simulink model "sm_dump_trailer"  (R2021b)
settings: Solver=VariableStepAuto  StartTime=0.0  StopTime=10  FixedStep=0.0001  RelTol=1e-3  AbsTol=1e-3  EnableMultiTasking=on
model workspace: external: MATLAB File sm_dump_trailer_params.m (data not in the file)
undefined symbols (not defined in the file or in its folder): base, bed, cylinder, lowerarm, sigbuilder_block, upperarm, X, Y, Z
libraries: sm_lib x65, sm_dump_trailer_lib x20, fl_lib x7, nesl_utility x4, simulink x4, sm_interface_elements_lib x1
(part 2 of 3)

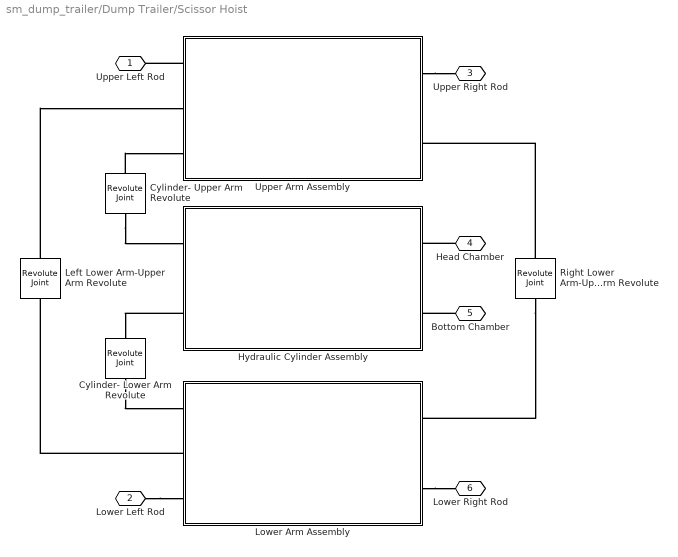
== system sm_dump_trailer/Dump Trailer/Scissor Hoist ==
  Cylinder- Lower Arm Revolute : sm_lib/Joints/Revolute Joint  JointMode=Normal  SenseConstraintForce=off  SenseConstraintForceX=off  SenseConstraintForceY=off  SenseConstraintForceZ=off  SenseConstraintTorque=off  SenseConstraintTorqueX=off  SenseConstraintTorqueY=off  SenseConstraintTorqueZ=off  SenseTotalForce=off  SenseTotalForceX=off  SenseTotalForceY=off  SenseTotalForceZ=off  SenseTotalTorque=off  SenseTotalTorqueX=off  SenseTotalTorqueY=off  SenseTotalTorqueZ=off  CompositeWrenchDir=FollowerOnBase  CompositeWrenchFrame=BaseFrame  EquilibriumPosition=0  EquilibriumPositionUnits=deg  SpringStiffness=0  SpringStiffnessUnits=N*m/deg  DampingCoefficient=0  DampingCoefficientUnits=N*m/(deg/s)  TorqueActuationMode=NoTorque  MotionActuationMode=ComputedMotion  SensePosition=off  SenseVelocity=off  SenseAcceleration=off  SenseTorqueForce=off  SenseLowerLimitTorqueForce=off  SenseUpperLimitTorqueForce=off  LowerLimitSpecify=off  LowerLimitBound=-90  LowerLimitBoundUnits=deg  LowerLimitStiffness=1e4  LowerLimitStiffnessUnits=N*m/deg  LowerLimitDamping=10  LowerLimitDampingUnits=N*m/(deg/s)  LowerLimitTransitionRegionWidth=0.1  LowerLimitTransitionRegionWidthUnits=deg  UpperLimitSpecify=off  UpperLimitBound=90  UpperLimitBoundUnits=deg  UpperLimitStiffness=1e4  UpperLimitStiffnessUnits=N*m/deg  UpperLimitDamping=10  UpperLimitDampingUnits=N*m/(deg/s)  UpperLimitTransitionRegionWidth=0.1  UpperLimitTransitionRegionWidthUnits=deg  PositionTargetSpecify=off  PositionTargetPriority=High  PositionTargetValue=0  PositionTargetValueUnits=deg  VelocityTargetSpecify=off  VelocityTargetPriority=High  VelocityTargetValue=0  VelocityTargetValueUnits=deg/s
  Cylinder- Upper Arm Revolute : sm_lib/Joints/Revolute Joint  JointMode=Normal  SenseConstraintForce=off  SenseConstraintForceX=off  SenseConstraintForceY=off  SenseConstraintForceZ=off  SenseConstraintTorque=off  SenseConstraintTorqueX=off  SenseConstraintTorqueY=off  SenseConstraintTorqueZ=off  SenseTotalForce=off  SenseTotalForceX=off  SenseTotalForceY=off  SenseTotalForceZ=off  SenseTotalTorque=off  SenseTotalTorqueX=off  SenseTotalTorqueY=off  SenseTotalTorqueZ=off  CompositeWrenchDir=FollowerOnBase  CompositeWrenchFrame=BaseFrame  EquilibriumPosition=0  EquilibriumPositionUnits=deg  SpringStiffness=0  SpringStiffnessUnits=N*m/deg  DampingCoefficient=0  DampingCoefficientUnits=N*m/(deg/s)  TorqueActuationMode=NoTorque  MotionActuationMode=ComputedMotion  SensePosition=off  SenseVelocity=off  SenseAcceleration=off  SenseTorqueForce=off  SenseLowerLimitTorqueForce=off  SenseUpperLimitTorqueForce=off  LowerLimitSpecify=off  LowerLimitBound=-90  LowerLimitBoundUnits=deg  LowerLimitStiffness=1e4  LowerLimitStiffnessUnits=N*m/deg  LowerLimitDamping=10  LowerLimitDampingUnits=N*m/(deg/s)  LowerLimitTransitionRegionWidth=0.1  LowerLimitTransitionRegionWidthUnits=deg  UpperLimitSpecify=off  UpperLimitBound=90  UpperLimitBoundUnits=deg  UpperLimitStiffness=1e4  UpperLimitStiffnessUnits=N*m/deg  UpperLimitDamping=10  UpperLimitDampingUnits=N*m/(deg/s)  UpperLimitTransitionRegionWidth=0.1  UpperLimitTransitionRegionWidthUnits=deg  PositionTargetSpecify=off  PositionTargetPriority=High  PositionTargetValue=0  PositionTargetValueUnits=deg  VelocityTargetSpecify=off  VelocityTargetPriority=High  VelocityTargetValue=0  VelocityTargetValueUnits=deg/s
  Hydraulic Cylinder Assembly : Subsystem
      mask Display: image(fullfile(matlabroot,'toolbox','physmod','sm','smdemos','dump_trailer','images','sm_dump_trailer_hydraulic_cylinder_assembly.png'));
  Left Lower Arm-Upper Arm Revolute : sm_lib/Joints/Revolute Joint  JointMode=Normal  SenseConstraintForce=off  SenseConstraintForceX=off  SenseConstraintForceY=off  SenseConstraintForceZ=off  SenseConstraintTorque=off  SenseConstraintTorqueX=off  SenseConstraintTorqueY=off  SenseConstraintTorqueZ=off  SenseTotalForce=off  SenseTotalForceX=off  SenseTotalForceY=off  SenseTotalForceZ=off  SenseTotalTorque=off  SenseTotalTorqueX=off  SenseTotalTorqueY=off  SenseTotalTorqueZ=off  CompositeWrenchDir=FollowerOnBase  CompositeWrenchFrame=BaseFrame  EquilibriumPosition=0  EquilibriumPositionUnits=deg  SpringStiffness=0  SpringStiffnessUnits=N*m/deg  DampingCoefficient=0  DampingCoefficientUnits=N*m/(deg/s)  TorqueActuationMode=NoTorque  MotionActuationMode=ComputedMotion  SensePosition=off  SenseVelocity=off  SenseAcceleration=off  SenseTorqueForce=off  SenseLowerLimitTorqueForce=off  SenseUpperLimitTorqueForce=off  LowerLimitSpecify=off  LowerLimitBound=-90  LowerLimitBoundUnits=deg  LowerLimitStiffness=1e4  LowerLimitStiffnessUnits=N*m/deg  LowerLimitDamping=10  LowerLimitDampingUnits=N*m/(deg/s)  LowerLimitTransitionRegionWidth=0.1  LowerLimitTransitionRegionWidthUnits=deg  UpperLimitSpecify=off  UpperLimitBound=90  UpperLimitBoundUnits=deg  UpperLimitStiffness=1e4  UpperLimitStiffnessUnits=N*m/deg  UpperLimitDamping=10  UpperLimitDampingUnits=N*m/(deg/s)  UpperLimitTransitionRegionWidth=0.1  UpperLimitTransitionRegionWidthUnits=deg  PositionTargetSpecify=off  PositionTargetPriority=High  PositionTargetValue=0  PositionTargetValueUnits=deg  VelocityTargetSpecify=off  VelocityTargetPriority=High  VelocityTargetValue=0  VelocityTargetValueUnits=deg/s
  Lower Arm Assembly : Subsystem
      mask Display: image(fullfile(matlabroot,'toolbox','physmod','sm','smdemos','dump_trailer','images','sm_dump_trailer_lower_arm_assembly.png'));
  Right Lower Arm-Upper Arm Revolute : sm_lib/Joints/Revolute Joint  JointMode=Normal  SenseConstraintForce=off  SenseConstraintForceX=off  SenseConstraintForceY=off  SenseConstraintForceZ=off  SenseConstraintTorque=off  SenseConstraintTorqueX=off  SenseConstraintTorqueY=off  SenseConstraintTorqueZ=off  SenseTotalForce=off  SenseTotalForceX=off  SenseTotalForceY=off  SenseTotalForceZ=off  SenseTotalTorque=off  SenseTotalTorqueX=off  SenseTotalTorqueY=off  SenseTotalTorqueZ=off  CompositeWrenchDir=FollowerOnBase  CompositeWrenchFrame=BaseFrame  EquilibriumPosition=0  EquilibriumPositionUnits=deg  SpringStiffness=0  SpringStiffnessUnits=N*m/deg  DampingCoefficient=0  DampingCoefficientUnits=N*m/(deg/s)  TorqueActuationMode=NoTorque  MotionActuationMode=ComputedMotion  SensePosition=off  SenseVelocity=off  SenseAcceleration=off  SenseTorqueForce=off  SenseLowerLimitTorqueForce=off  SenseUpperLimitTorqueForce=off  LowerLimitSpecify=off  LowerLimitBound=-90  LowerLimitBoundUnits=deg  LowerLimitStiffness=1e4  LowerLimitStiffnessUnits=N*m/deg  LowerLimitDamping=10  LowerLimitDampingUnits=N*m/(deg/s)  LowerLimitTransitionRegionWidth=0.1  LowerLimitTransitionRegionWidthUnits=deg  UpperLimitSpecify=off  UpperLimitBound=90  UpperLimitBoundUnits=deg  UpperLimitStiffness=1e4  UpperLimitStiffnessUnits=N*m/deg  UpperLimitDamping=10  UpperLimitDampingUnits=N*m/(deg/s)  UpperLimitTransitionRegionWidth=0.1  UpperLimitTransitionRegionWidthUnits=deg  PositionTargetSpecify=off  PositionTargetPriority=High  PositionTargetValue=0  PositionTargetValueUnits=deg  VelocityTargetSpecify=off  VelocityTargetPriority=High  VelocityTargetValue=0  VelocityTargetValueUnits=deg/s
  Upper Arm Assembly : Subsystem
      mask Display: image(fullfile(matlabroot,'toolbox','physmod','sm','smdemos','dump_trailer','images','sm_dump_trailer_upper_arm_assembly.png'));
  Upper Left Rod : PMIOPort  Side=Left
  Lower Left Rod : PMIOPort  Port=2  Side=Left
  Upper Right Rod : PMIOPort  Port=3  Side=Right
  Head Chamber : PMIOPort  Port=4  Side=Right
  Bottom Chamber : PMIOPort  Port=5  Side=Right
  Lower Right Rod : PMIOPort  Port=6  Side=Right
  connections:
  Right Lower Arm-Upper Arm Revolute/LConn1 -- Lower Arm Assembly/RConn1
  Lower Arm Assembly/LConn2 -- Left Lower Arm-Upper Arm Revolute/LConn1
  Upper Arm Assembly/LConn1 -- Upper Left Rod/RConn1
  Upper Arm Assembly/RConn1 -- Upper Right Rod/RConn1
  Lower Arm Assembly/RConn2 -- Lower Right Rod/RConn1
  Left Lower Arm-Upper Arm Revolute/RConn1 -- Upper Arm Assembly/LConn2
  Right Lower Arm-Upper Arm Revolute/RConn1 -- Upper Arm Assembly/RConn2
  Lower Left Rod/RConn1 -- Lower Arm Assembly/LConn3
  Head Chamber/RConn1 -- Hydraulic Cylinder Assembly/RConn1
  Bottom Chamber/RConn1 -- Hydraulic Cylinder Assembly/RConn2
  Cylinder- Lower Arm Revolute/LConn1 -- Lower Arm Assembly/LConn1
  Hydraulic Cylinder Assembly/LConn2 -- Cylinder- Lower Arm Revolute/RConn1
  Cylinder- Upper Arm Revolute/LConn1 -- Hydraulic Cylinder Assembly/LConn1
  Cylinder- Upper Arm Revolute/RConn1 -- Upper Arm Assembly/LConn3

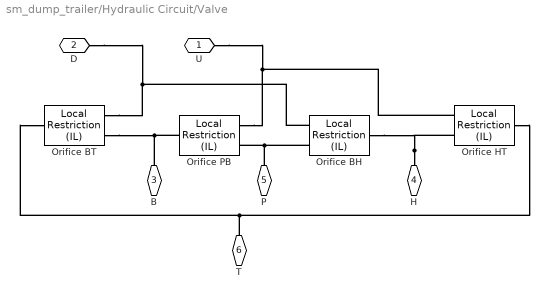
== system sm_dump_trailer/Hydraulic Circuit/Valve ==
  Orifice BH : fl_lib/Isothermal Liquid/Elements/Local Restriction (IL)  restriction_type=foundation.enum.restriction_type.variable  restriction_area=1e-3 m^2  min_area=1e-12 m^2  max_area=2.5e-5 m^2  area=inf m^2  Cd=0.7  Re_c=150  pressure_recovery=simscape.enum.onoff.off
      settings: SourceProductBaseCode=SS  InternalSimscapePortConfiguration="{\"Bottom\":[],\"Left\":[{\"id\":\"A\",\"label\":\"A\",\"type\":\"foundation.isothermal_liquid.isothermal_liquid\"},{\"id\":\"AR\",\"label\":\"AR\",\"type\":\"input\"}],\"Right\":[{\"id\":\"B\",\"label\":\"B\",\"type\":\"foundation.isothermal_liquid.isothermal_liquid\"}],\"Top\":[]}"
  Orifice BT : fl_lib/Isothermal Liquid/Elements/Local Restriction (IL)  restriction_type=foundation.enum.restriction_type.variable  restriction_area=1e-3 m^2  min_area=1e-12 m^2  max_area=2.5e-5 m^2  area=inf m^2  Cd=0.7  Re_c=150  pressure_recovery=simscape.enum.onoff.off
      settings: SourceProductBaseCode=SS  InternalSimscapePortConfiguration="{\"Bottom\":[],\"Left\":[{\"id\":\"A\",\"label\":\"A\",\"type\":\"foundation.isothermal_liquid.isothermal_liquid\"},{\"id\":\"AR\",\"label\":\"AR\",\"type\":\"input\"}],\"Right\":[{\"id\":\"B\",\"label\":\"B\",\"type\":\"foundation.isothermal_liquid.isothermal_liquid\"}],\"Top\":[]}"
  Orifice HT : fl_lib/Isothermal Liquid/Elements/Local Restriction (IL)  restriction_type=foundation.enum.restriction_type.variable  restriction_area=1e-3 m^2  min_area=1e-12 m^2  max_area=2.5e-5 m^2  area=inf m^2  Cd=0.7  Re_c=150  pressure_recovery=simscape.enum.onoff.off
      settings: SourceProductBaseCode=SS  InternalSimscapePortConfiguration="{\"Bottom\":[],\"Left\":[{\"id\":\"A\",\"label\":\"A\",\"type\":\"foundation.isothermal_liquid.isothermal_liquid\"},{\"id\":\"AR\",\"label\":\"AR\",\"type\":\"input\"}],\"Right\":[{\"id\":\"B\",\"label\":\"B\",\"type\":\"foundation.isothermal_liquid.isothermal_liquid\"}],\"Top\":[]}"
  Orifice PB : fl_lib/Isothermal Liquid/Elements/Local Restriction (IL)  restriction_type=foundation.enum.restriction_type.variable  restriction_area=1e-3 m^2  min_area=1e-12 m^2  max_area=2.5e-5 m^2  area=inf m^2  Cd=0.7  Re_c=150  pressure_recovery=simscape.enum.onoff.off
      settings: SourceProductBaseCode=SS  InternalSimscapePortConfiguration="{\"Bottom\":[],\"Left\":[{\"id\":\"A\",\"label\":\"A\",\"type\":\"foundation.isothermal_liquid.isothermal_liquid\"},{\"id\":\"AR\",\"label\":\"AR\",\"type\":\"input\"}],\"Right\":[{\"id\":\"B\",\"label\":\"B\",\"type\":\"foundation.isothermal_liquid.isothermal_liquid\"}],\"Top\":[]}"
  U : PMIOPort  Side=Left
  D : PMIOPort  Port=2  Side=Left
  B : PMIOPort  Port=3  Side=Right
  H : PMIOPort  Port=4  Side=Right
  P : PMIOPort  Port=5  Side=Left
  T : PMIOPort  Port=6  Side=Left
  connections:
  Orifice BH/LConn1 -- P/RConn1 -- Orifice PB/LConn1
  Orifice HT/RConn1 -- T/RConn1 -- Orifice BT/RConn1
  U/RConn1 -- Orifice PB/LConn2 -- Orifice HT/LConn2
  D/RConn1 -- Orifice BT/LConn2 -- Orifice BH/LConn2
  B/RConn1 -- Orifice BT/LConn1 -- Orifice PB/RConn1
  H/RConn1 -- Orifice HT/LConn1 -- Orifice BH/RConn1

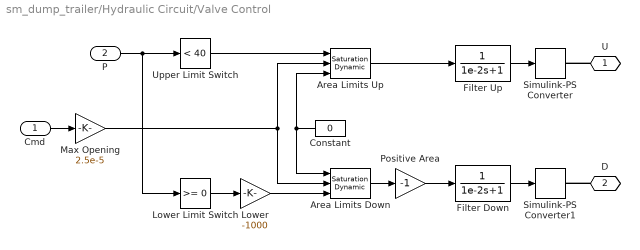
== system sm_dump_trailer/Hydraulic Circuit/Valve Control ==
  Cmd : Inport
  P : Inport  Port=2
  Area Limits Down : simulink/Discontinuities/Saturation Dynamic  OutMin=[]  OutMax=[]  OutDataTypeStr=Inherit: Same as second input  OutDataType=fixdt(1, 16)  OutScaling=2^-10  DoSatur=off
  Area Limits Up : simulink/Discontinuities/Saturation Dynamic  OutMin=[]  OutMax=[]  OutDataTypeStr=Inherit: Same as second input  OutDataType=fixdt(1, 16)  OutScaling=2^-10  DoSatur=off
  Constant : Constant  Value=0
  Filter Down : TransferFcn  Denominator=[1e-2 1]
  Filter Up : TransferFcn  Denominator=[1e-2 1]
  Lower : Gain  Gain=-1000
  Lower Limit Switch : simulink/Logic and Bit Operations/Compare To Constant  relop=>=  const=0  OutDataTypeStr=boolean
  Max Opening : Gain  Gain=2.5e-5
  Positive Area : Gain  Gain=-1
  Simulink-PS Converter : nesl_utility/Simulink-PS Converter  PhysicalDomain=network_engine_domain  SubClassName=ps_input  LeftPortType=input  RightPortType=output  PseudoPeriodic=off  Frequencies=[]  NoiseDistribution=none  NoiseParameters=[]  Unit=1  AffineConversion=off  FilteringAndDerivatives=zero  SimscapeFilterOrder=1  InputFilterTimeConstant=0.001  UdotUserProvided=1
      settings: SourceProductBaseCode=PW,SS
  Simulink-PS Converter1 : nesl_utility/Simulink-PS Converter  PhysicalDomain=network_engine_domain  SubClassName=ps_input  LeftPortType=input  RightPortType=output  PseudoPeriodic=off  Frequencies=[]  NoiseDistribution=none  NoiseParameters=[]  Unit=1  AffineConversion=off  FilteringAndDerivatives=zero  SimscapeFilterOrder=1  InputFilterTimeConstant=0.001  UdotUserProvided=1
      settings: SourceProductBaseCode=PW,SS
  Upper Limit Switch : simulink/Logic and Bit Operations/Compare To Constant  relop=<  const=40  OutDataTypeStr=boolean
  U : PMIOPort  Side=Right
  D : PMIOPort  Port=2  Side=Right
  wires:
  Cmd/1 -> Max Opening/1
  Area Limits Down/1 -> Positive Area/1
  Area Limits Up/1 -> Filter Up/1
  Positive Area/1 -> Filter Down/1
  Max Opening/1 -> Area Limits Up/2, Area Limits Down/2
  Filter Up/1 -> Simulink-PS Converter/1
  Filter Down/1 -> Simulink-PS Converter1/1
  Constant/1 -> Area Limits Down/1, Area Limits Up/3
  P/1 -> Lower Limit Switch/1, Upper Limit Switch/1
  Upper Limit Switch/1 -> Area Limits Up/1
  Lower Limit Switch/1 -> Lower/1
  Lower/1 -> Area Limits Down/3
  connections:
  U/RConn1 -- Simulink-PS Converter/RConn1
  D/RConn1 -- Simulink-PS Converter1/RConn1

== system sm_dump_trailer/Dump Trailer/Base Assembly/Hitch ==
  Ball : sm_lib/Body Elements/Spherical Solid  GraphicAmbientColor=[0.15 0.15 0.15 1.0]  BasedOnType=Density  CenterOfMass=[0 0 0]  CenterOfMassUnits=m  GraphicDiffuseColor=color_ball  Density=rho_ball  DensityUnits=kg/m^3  DoExposeReferenceFrame=on  GraphicEmissiveColor=[0.0 0.0 0.0 1.0]  ExportEntireGeometry=off  SerializedExposedGeometries=<ExposedGeometries/>  SerializedFrames=<Frames/>  MarkerShape=Sphere  MarkerSize=10  GraphicType=FromGeometry  InertiaType=CalculateFromGeometry  Mass=1  MassUnits=kg  MomentsOfInertia=[1 1 1]  MomentsOfInertiaUnits=kg*m^2  GraphicOpacity=1.0  ProductsOfInertia=[1 1 1]  ProductsOfInertiaUnits=kg*m^2  GraphicShininess=75  GraphicSpecularColor=[0.5 0.5 0.5 1.0]  SphereRadius=r_ball  SphereRadiusUnits=m  GraphicVisPropType=SimpleVisualProperties
  Bar : sm_lib/Body Elements/Brick Solid  GraphicAmbientColor=[0.15 0.15 0.15 1.0]  BasedOnType=Density  BrickDimensions=[L_bar W_bar H_bar]  BrickDimensionUnits=m  CenterOfMass=[0 0 0]  CenterOfMassUnits=m  GraphicDiffuseColor=color_bar  Density=rho_bar  DensityUnits=kg/m^3  DoExposeReferenceFrame=off  GraphicEmissiveColor=[0.0 0.0 0.0 1.0]  ExportEntireGeometry=off  SerializedFrames=<Frames><Frame><Id>Frame1</Id><Value><Name>End</Name><Origin><Source>GeometricFeature</Source><FeatureName>+x surface</FeatureName></Origin><PrimaryAxis><DefinedDirection>+Y</DefinedDirection><Source>ReferenceFrame</Source><SourceDirection>+X</SourceDirection><FeatureName></FeatureName></PrimaryAxis><SecondaryAxis><DefinedDirection>+X</DefinedDirection><Source>ReferenceFrame</Source><SourceDirection>-Y</SourceDirection><FeatureName></FeatureName></SecondaryAxis></Value></Frame></Frames>  MarkerShape=Sphere  MarkerSize=10  GraphicType=FromGeometry  InertiaType=CalculateFromGeometry  Mass=1  MassUnits=kg  MomentsOfInertia=[1 1 1]  MomentsOfInertiaUnits=kg*m^2  GraphicOpacity=1.0  ProductsOfInertia=[1 1 1]  ProductsOfInertiaUnits=kg*m^2  GraphicShininess=75  GraphicSpecularColor=[0.5 0.5 0.5 1.0]  GraphicVisPropType=SimpleVisualProperties
  Cylinder : sm_lib/Body Elements/Cylindrical Solid  GraphicAmbientColor=[0.15 0.15 0.15 1.0]  BasedOnType=Density  CenterOfMass=[0 0 0]  CenterOfMassUnits=m  GraphicDiffuseColor=color_cyl  CylinderLength=L_cyl  CylinderLengthUnits=m  CylinderRadius=r_cyl  CylinderRadiusUnits=m  Density=rho_cyl  DensityUnits=kg/m^3  DoExposeReferenceFrame=on  GraphicEmissiveColor=[0.0 0.0 0.0 1.0]  ExportEntireGeometry=off  SerializedFrames=<Frames><Frame><Id>Frame1</Id><Value><Name>Top</Name><Origin><Source>GeometricFeature</Source><FeatureName>top surface</FeatureName></Origin><PrimaryAxis><DefinedDirection>+Z</DefinedDirection><Source>ReferenceFrame</Source><SourceDirection>+Z</SourceDirection><FeatureName></FeatureName></PrimaryAxis><SecondaryAxis><DefinedDirection>+X</DefinedDirection><Source>ReferenceFrame</Source><SourceDirection>+X</SourceDirection><FeatureName></FeatureName></SecondaryAxis></Value></Frame></Frames>  MarkerShape=Sphere  MarkerSize=10  GraphicType=FromGeometry  InertiaType=CalculateFromGeometry  Mass=1  MassUnits=kg  MomentsOfInertia=[1 1 1]  MomentsOfInertiaUnits=kg*m^2  GraphicOpacity=1.0  ProductsOfInertia=[1 1 1]  ProductsOfInertiaUnits=kg*m^2  GraphicShininess=75  GraphicSpecularColor=[0.5 0.5 0.5 1.0]  GraphicVisPropType=SimpleVisualProperties
  Cylinder XForm : sm_lib/Frames and Transforms/Rigid Transform  TranslationMethod=Cartesian  TranslationStandardOffset=0  TranslationLengthUnit=m  TranslationStandardAxis=-Y  TranslationCartesianOffset=base.hitch.cylinder.offset  TranslationROffset=0  TranslationROffsetUnits=m  TranslationZOffset=0  TranslationZOffsetUnits=m  TranslationThetaOffset=0  TranslationThetaOffsetUnits=deg  RotationMethod=None  RotationAngleUnits=deg  RotationStandardAxis=-Z  RotationAngle=90  RotationArbitraryAxis=[0 0 1]  FollAlignAxisA=+X  BaseAlignAxisA=+Y  FollAlignAxisB=+Y  BaseAlignAxisB=+Z  RotationSequenceAxes=FollowerAxes  RotationSequence=XYX  RotationSequenceAngles=[0 0 0]  RotationSequenceAnglesUnits=deg  RotationMatrix=[1 0 0; 0 1 0; 0 0 1]
  "Frame " : PMIOPort  Side=Left
  Hitch : PMIOPort  Port=2  Side=Right
  connections:
  Cylinder XForm/RConn1 -- Cylinder/RConn1
  Bar/LConn1 -- "Frame "/RConn1 -- Cylinder XForm/LConn1
  Ball/RConn1 -- Hitch/RConn1 -- Cylinder/LConn1

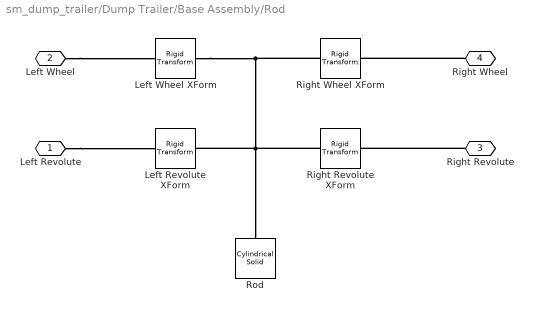
== system sm_dump_trailer/Dump Trailer/Base Assembly/Rod ==
  Left Revolute XForm : sm_lib/Frames and Transforms/Rigid Transform  TranslationMethod=StandardAxis  TranslationStandardOffset=d_rev  TranslationLengthUnit=m  TranslationStandardAxis=-Z  TranslationCartesianOffset=[0 0 0]  TranslationROffset=0  TranslationROffsetUnits=m  TranslationZOffset=0  TranslationZOffsetUnits=m  TranslationThetaOffset=0  TranslationThetaOffsetUnits=deg  RotationMethod=None  RotationAngleUnits=deg  RotationStandardAxis=+Z  RotationAngle=0.0  RotationArbitraryAxis=[0 0 1]  FollAlignAxisA=+X  BaseAlignAxisA=+Y  FollAlignAxisB=+Y  BaseAlignAxisB=+Z  RotationSequenceAxes=FollowerAxes  RotationSequence=XYX  RotationSequenceAngles=[0 0 0]  RotationSequenceAnglesUnits=deg  RotationMatrix=[1 0 0; 0 1 0; 0 0 1]
  Left Wheel XForm : sm_lib/Frames and Transforms/Rigid Transform  TranslationMethod=StandardAxis  TranslationStandardOffset=d_wheel  TranslationLengthUnit=m  TranslationStandardAxis=-Z  TranslationCartesianOffset=[0 0 0]  TranslationROffset=0  TranslationROffsetUnits=m  TranslationZOffset=0  TranslationZOffsetUnits=m  TranslationThetaOffset=0  TranslationThetaOffsetUnits=deg  RotationMethod=None  RotationAngleUnits=deg  RotationStandardAxis=+Z  RotationAngle=0.0  RotationArbitraryAxis=[0 0 1]  FollAlignAxisA=+Z  BaseAlignAxisA=-Z  FollAlignAxisB=+Y  BaseAlignAxisB=+Y  RotationSequenceAxes=FollowerAxes  RotationSequence=XYX  RotationSequenceAngles=[0 0 0]  RotationSequenceAnglesUnits=deg  RotationMatrix=[1 0 0; 0 1 0; 0 0 1]
  Right Revolute XForm : sm_lib/Frames and Transforms/Rigid Transform  TranslationMethod=StandardAxis  TranslationStandardOffset=d_rev  TranslationLengthUnit=m  TranslationStandardAxis=+Z  TranslationCartesianOffset=[0 0 0]  TranslationROffset=0  TranslationROffsetUnits=m  TranslationZOffset=0  TranslationZOffsetUnits=m  TranslationThetaOffset=0  TranslationThetaOffsetUnits=deg  RotationMethod=None  RotationAngleUnits=deg  RotationStandardAxis=+Z  RotationAngle=0.0  RotationArbitraryAxis=[0 0 1]  FollAlignAxisA=+X  BaseAlignAxisA=+Y  FollAlignAxisB=+Y  BaseAlignAxisB=+Z  RotationSequenceAxes=FollowerAxes  RotationSequence=XYX  RotationSequenceAngles=[0 0 0]  RotationSequenceAnglesUnits=deg  RotationMatrix=[1 0 0; 0 1 0; 0 0 1]
  Right Wheel XForm : sm_lib/Frames and Transforms/Rigid Transform  TranslationMethod=StandardAxis  TranslationStandardOffset=d_wheel  TranslationLengthUnit=m  TranslationStandardAxis=+Z  TranslationCartesianOffset=[0 0 0]  TranslationROffset=0  TranslationROffsetUnits=m  TranslationZOffset=0  TranslationZOffsetUnits=m  TranslationThetaOffset=0  TranslationThetaOffsetUnits=deg  RotationMethod=None  RotationAngleUnits=deg  RotationStandardAxis=+Y  RotationAngle=180  RotationArbitraryAxis=[0 0 1]  FollAlignAxisA=+Z  BaseAlignAxisA=-Z  FollAlignAxisB=+Y  BaseAlignAxisB=+Y  RotationSequenceAxes=FollowerAxes  RotationSequence=YZX  RotationSequenceAngles=[180 180 0]  RotationSequenceAnglesUnits=deg  RotationMatrix=[1 0 0; 0 1 0; 0 0 1]
  Rod : sm_lib/Body Elements/Cylindrical Solid  GraphicAmbientColor=[0.15 0.15 0.15 1.0]  BasedOnType=Density  CenterOfMass=[0 0 0]  CenterOfMassUnits=m  GraphicDiffuseColor=color  CylinderLength=L  CylinderLengthUnits=m  CylinderRadius=r  CylinderRadiusUnits=m  Density=rho  DensityUnits=kg/m^3  DoExposeReferenceFrame=on  GraphicEmissiveColor=[0.0 0.0 0.0 1.0]  ExportEntireGeometry=off  SerializedFrames=<Frames/>  MarkerShape=Sphere  MarkerSize=10  GraphicType=FromGeometry  InertiaType=CalculateFromGeometry  Mass=1  MassUnits=kg  MomentsOfInertia=[1 1 1]  MomentsOfInertiaUnits=kg*m^2  GraphicOpacity=1.0  ProductsOfInertia=[1 1 1]  ProductsOfInertiaUnits=kg*m^2  GraphicShininess=75  GraphicSpecularColor=[0.5 0.5 0.5 1.0]  GraphicVisPropType=SimpleVisualProperties
  Left Revolute : PMIOPort  Side=Left
  Left Wheel : PMIOPort  Port=2  Side=Left
  Right Revolute : PMIOPort  Port=3  Side=Right
  Right Wheel : PMIOPort  Port=4  Side=Right
  connections:
  Right Wheel XForm/LConn1 -- Left Revolute XForm/LConn1 -- Rod/RConn1 -- Right Revolute XForm/LConn1 -- Left Wheel XForm/LConn1
  Left Wheel/RConn1 -- Left Wheel XForm/RConn1
  Left Revolute/RConn1 -- Left Revolute XForm/RConn1
  Right Wheel/RConn1 -- Right Wheel XForm/RConn1
  Right Revolute/RConn1 -- Right Revolute XForm/RConn1

== system sm_dump_trailer/Dump Trailer/Bed Assembly/Bed ==
  Floor : sm_lib/Body Elements/Brick Solid  GraphicAmbientColor=[0.15 0.15 0.15 1.0]  BasedOnType=Density  BrickDimensions=[L W T_floor]  BrickDimensionUnits=m  CenterOfMass=[0 0 0]  CenterOfMassUnits=m  GraphicDiffuseColor=color_floor  Density=rho_floor  DensityUnits=kg/m^3  DoExposeReferenceFrame=on  GraphicEmissiveColor=[0.0 0.0 0.0 1.0]  ExportEntireGeometry=off  SerializedFrames=<Frames><Frame><Id>Frame1</Id><Value><Name>top</Name><Origin><Source>GeometricFeature</Source><FeatureName>+z +x curve</FeatureName></Origin><PrimaryAxis><DefinedDirection>+Z</DefinedDirection><Source>ReferenceFrame</Source><SourceDirection>+Z</SourceDirection><FeatureName></FeatureName></PrimaryAxis><SecondaryAxis><DefinedDirection>+X</DefinedDirection><Source>ReferenceFrame</Source><SourceDirection>+X</SourceDirection><FeatureName></FeatureName></SecondaryAxis></Value></Frame></Frames>  MarkerShape=Sphere  MarkerSize=10  GraphicType=FromGeometry  InertiaType=CalculateFromGeometry  Mass=1  MassUnits=kg  MomentsOfInertia=[1 1 1]  MomentsOfInertiaUnits=kg*m^2  GraphicOpacity=1.0  ProductsOfInertia=[1 1 1]  ProductsOfInertiaUnits=kg*m^2  GraphicShininess=75  GraphicSpecularColor=[0.5 0.5 0.5 1.0]  GraphicVisPropType=SimpleVisualProperties
  Wall : sm_lib/Body Elements/Extruded Solid  GraphicAmbientColor=[0.15 0.15 0.15 1.0]  BasedOnType=Density  CenterOfMass=[0 0 0]  CenterOfMassUnits=m  GraphicDiffuseColor=color_wall  ExportConvexHullGeometry=off  ExtrusionCrossSection=CS  ExtrusionCrossSectionUnits=m  Density=rho_wall  DensityUnits=kg/m^3  DoExposeReferenceFrame=off  GraphicEmissiveColor=[0.0 0.0 0.0 1.0]  ExportEntireGeometry=off  ExtrusionLength=H  ExtrusionLengthUnits=m  ExtrusionType=General  SerializedFrames=<Frames><Frame><Id>Frame1</Id><Value><Name>bottom</Name><Origin><Source>GeometricFeature</Source><FeatureName>bottom curve 20</FeatureName></Origin><PrimaryAxis><DefinedDirection>+Z</DefinedDirection><Source>ReferenceFrame</Source><SourceDirection>+Z</SourceDirection><FeatureName></FeatureName></PrimaryAxis><SecondaryAxis><DefinedDirection>+X</DefinedDirection><Source>ReferenceFrame</Source><SourceDirection>+X</SourceDirection><FeatureName></FeatureName></SecondaryAxis></Value></Frame></Frames>  MarkerShape=Sphere  MarkerSize=10  GraphicType=FromGeometry  InertiaType=CalculateFromGeometry  Mass=1  MassUnits=kg  MomentsOfInertia=[1 1 1]  MomentsOfInertiaUnits=kg*m^2  PolygonNumSides=3  GraphicOpacity=1.0  PolygonOuterRadius=1  PolygonOuterRadiusUnits=m  ProductsOfInertia=[1 1 1]  ProductsOfInertiaUnits=kg*m^2  GraphicShininess=75  GraphicSpecularColor=[0.5 0.5 0.5 1]  GraphicVisPropType=SimpleVisualProperties
  Center : PMIOPort  Side=Right
  connections:
  Floor/RConn1 -- Center/RConn1
  Wall/LConn1 -- Floor/LConn1

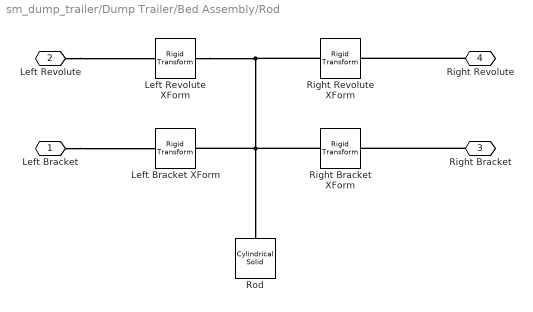
== system sm_dump_trailer/Dump Trailer/Bed Assembly/Rod ==
  Left Bracket XForm : sm_lib/Frames and Transforms/Rigid Transform  TranslationMethod=StandardAxis  TranslationStandardOffset=d_bracket  TranslationLengthUnit=m  TranslationStandardAxis=-Z  TranslationCartesianOffset=[0 0 0]  TranslationROffset=0  TranslationROffsetUnits=m  TranslationZOffset=0  TranslationZOffsetUnits=m  TranslationThetaOffset=0  TranslationThetaOffsetUnits=deg  RotationMethod=None  RotationAngleUnits=deg  RotationStandardAxis=+Z  RotationAngle=0.0  RotationArbitraryAxis=[0 0 1]  FollAlignAxisA=+X  BaseAlignAxisA=+Y  FollAlignAxisB=+Y  BaseAlignAxisB=+Z  RotationSequenceAxes=FollowerAxes  RotationSequence=XYX  RotationSequenceAngles=[0 0 0]  RotationSequenceAnglesUnits=deg  RotationMatrix=[1 0 0; 0 1 0; 0 0 1]
  Left Revolute XForm : sm_lib/Frames and Transforms/Rigid Transform  TranslationMethod=StandardAxis  TranslationStandardOffset=d_rev  TranslationLengthUnit=m  TranslationStandardAxis=-Z  TranslationCartesianOffset=[0 0 0]  TranslationROffset=0  TranslationROffsetUnits=m  TranslationZOffset=0  TranslationZOffsetUnits=m  TranslationThetaOffset=0  TranslationThetaOffsetUnits=deg  RotationMethod=None  RotationAngleUnits=deg  RotationStandardAxis=+Z  RotationAngle=0.0  RotationArbitraryAxis=[0 0 1]  FollAlignAxisA=+Z  BaseAlignAxisA=-Z  FollAlignAxisB=+Y  BaseAlignAxisB=+Y  RotationSequenceAxes=FollowerAxes  RotationSequence=XYX  RotationSequenceAngles=[0 0 0]  RotationSequenceAnglesUnits=deg  RotationMatrix=[1 0 0; 0 1 0; 0 0 1]
  Right Bracket XForm : sm_lib/Frames and Transforms/Rigid Transform  TranslationMethod=StandardAxis  TranslationStandardOffset=d_bracket  TranslationLengthUnit=m  TranslationStandardAxis=+Z  TranslationCartesianOffset=[0 0 0]  TranslationROffset=0  TranslationROffsetUnits=m  TranslationZOffset=0  TranslationZOffsetUnits=m  TranslationThetaOffset=0  TranslationThetaOffsetUnits=deg  RotationMethod=None  RotationAngleUnits=deg  RotationStandardAxis=+Z  RotationAngle=0.0  RotationArbitraryAxis=[0 0 1]  FollAlignAxisA=+X  BaseAlignAxisA=+Y  FollAlignAxisB=+Y  BaseAlignAxisB=+Z  RotationSequenceAxes=FollowerAxes  RotationSequence=XYX  RotationSequenceAngles=[0 0 0]  RotationSequenceAnglesUnits=deg  RotationMatrix=[1 0 0; 0 1 0; 0 0 1]
  Right Revolute XForm : sm_lib/Frames and Transforms/Rigid Transform  TranslationMethod=StandardAxis  TranslationStandardOffset=d_rev  TranslationLengthUnit=m  TranslationStandardAxis=+Z  TranslationCartesianOffset=[0 0 0]  TranslationROffset=0  TranslationROffsetUnits=m  TranslationZOffset=0  TranslationZOffsetUnits=m  TranslationThetaOffset=0  TranslationThetaOffsetUnits=deg  RotationMethod=RotationSequence  RotationAngleUnits=deg  RotationStandardAxis=+Y  RotationAngle=180  RotationArbitraryAxis=[0 0 1]  FollAlignAxisA=+Z  BaseAlignAxisA=-Z  FollAlignAxisB=+Y  BaseAlignAxisB=+Y  RotationSequenceAxes=FollowerAxes  RotationSequence=YZX  RotationSequenceAngles=[180 180 0]  RotationSequenceAnglesUnits=deg  RotationMatrix=[1 0 0; 0 1 0; 0 0 1]
  Rod : sm_lib/Body Elements/Cylindrical Solid  GraphicAmbientColor=[0.15 0.15 0.15 1.0]  BasedOnType=Density  CenterOfMass=[0 0 0]  CenterOfMassUnits=m  GraphicDiffuseColor=color  CylinderLength=L  CylinderLengthUnits=m  CylinderRadius=r  CylinderRadiusUnits=m  Density=rho  DensityUnits=kg/m^3  DoExposeReferenceFrame=on  GraphicEmissiveColor=[0.0 0.0 0.0 1.0]  ExportEntireGeometry=off  SerializedFrames=<Frames/>  MarkerShape=Sphere  MarkerSize=10  GraphicType=FromGeometry  InertiaType=CalculateFromGeometry  Mass=1  MassUnits=kg  MomentsOfInertia=[1 1 1]  MomentsOfInertiaUnits=kg*m^2  GraphicOpacity=1.0  ProductsOfInertia=[1 1 1]  ProductsOfInertiaUnits=kg*m^2  GraphicShininess=75  GraphicSpecularColor=[0.5 0.5 0.5 1.0]  GraphicVisPropType=SimpleVisualProperties
  Left Bracket : PMIOPort  Side=Left
  Left Revolute : PMIOPort  Port=2  Side=Left
  Right Bracket : PMIOPort  Port=3  Side=Right
  Right Revolute : PMIOPort  Port=4  Side=Right
  connections:
  Right Revolute XForm/LConn1 -- Left Bracket XForm/LConn1 -- Rod/RConn1 -- Right Bracket XForm/LConn1 -- Left Revolute XForm/LConn1
  Left Revolute/RConn1 -- Left Revolute XForm/RConn1
  Left Bracket/RConn1 -- Left Bracket XForm/RConn1
  Right Revolute/RConn1 -- Right Revolute XForm/RConn1
  Right Bracket/RConn1 -- Right Bracket XForm/RConn1

== system sm_dump_trailer/Dump Trailer/Scissor Hoist/Hydraulic Cylinder Assembly ==
  Bottom Bracket : sm_dump_trailer_lib/Bracket  Hbracket=cylinder.bottombracket.height  Wbracket=cylinder.bottombracket.width  Tbracket=cylinder.bottombracket.thickness  Hhole=cylinder.bottombracket.holeheight  Rhole=cylinder.bottombracket.holeradius  rho=cylinder.bottombracket.density  bracketColor=cylinder.bottombracket.color
      settings: SourceProductBaseCode=MS
  Double-Acting Hydraulic Cylinder : sm_interface_elements_lib/Hydraulic/Double-Acting Hydraulic Cylinder  barrelLength=cylinder.barrel.length  barrelInnerRadius=cylinder.barrel.innerradius  barrelOuterRadius=cylinder.barrel.outerradius  barrelDensity=cylinder.barrel.density  barrelColor=cylinder.barrel.color  barrelOpacity=cylinder.barrel.opacity  pistonThickness=cylinder.piston.thickness  pistonDensity=cylinder.piston.density  pistonColor=cylinder.piston.color  rodLength=cylinder.rod.length  rodRadius=cylinder.rod.radius  rodDensity=cylinder.rod.density  rodColor=cylinder.rod.color  bottomCapThickness=cylinder.bottomcap.thickness  bottomCapDensity=cylinder.bottomcap.density  bottomCapColor=cylinder.bottomcap.color  headCapThickness=cylinder.headcap.thickness  headCapDensity=cylinder.headcap.density  headCapColor=cylinder.headcap.color  deadVolume_bottom=cylinder.bottomchamber.deadvolume  deadVolume_head=cylinder.headchamber.deadvolume  k_bottom=cylinder.bottomstop.stiffness  b_bottom=cylinder.bottomstop.damping  k_head=cylinder.headstop.stiffness  b_head=cylinder.headstop.damping  b=cylinder.viscousdamping  PositionTargetSpecify=on  PositionTargetPriority=Low (approximate)  totalLength0=cylinder.endtoenddistance  p0_bottom=cylinder.bottomchamber.initialpressure  p0_head=cylinder.headchamber.initialpressure
      settings: SourceProductBaseCode=MS
  Top Bracket : sm_dump_trailer_lib/Bracket  Hbracket=cylinder.topbracket.height  Wbracket=cylinder.topbracket.width  Tbracket=cylinder.topbracket.thickness  Hhole=cylinder.topbracket.holeheight  Rhole=cylinder.topbracket.holeradius  rho=cylinder.topbracket.density  bracketColor=cylinder.topbracket.color
      settings: SourceProductBaseCode=MS
  Top Hole : PMIOPort  Side=Left
  Bottom Hole : PMIOPort  Port=2  Side=Left
  Head Chamber : PMIOPort  Port=3  Side=Right
  Bottom Chamber : PMIOPort  Port=4  Side=Right
  connections:
  Top Hole/RConn1 -- Top Bracket/RConn1
  Bottom Bracket/RConn1 -- Bottom Hole/RConn1
  Double-Acting Hydraulic Cylinder/LConn1 -- Bottom Bracket/LConn1
  Double-Acting Hydraulic Cylinder/RConn1 -- Top Bracket/LConn1
  Bottom Chamber/RConn1 -- Double-Acting Hydraulic Cylinder/LConn2
  Head Chamber/RConn1 -- Double-Acting Hydraulic Cylinder/RConn2

== system sm_dump_trailer/Dump Trailer/Scissor Hoist/Lower Arm Assembly ==
  Left Arm : sm_dump_trailer_lib/Lower Arm  L=lowerarm.length  H=lowerarm.height  T=lowerarm.thickness  d_h2h=lowerarm.hole2holedistance  r_h=lowerarm.holeradius  rho=lowerarm.density  color=lowerarm.color
      settings: SourceProductBaseCode=MS
  Right Arm : sm_dump_trailer_lib/Lower Arm  L=lowerarm.length  H=lowerarm.height  T=lowerarm.thickness  d_h2h=lowerarm.hole2holedistance  r_h=lowerarm.holeradius  rho=lowerarm.density  color=lowerarm.color
      settings: SourceProductBaseCode=MS
  Rod : Subsystem  mask{L=lowerarm.rod.length, r=lowerarm.rod.radius, d_arm=lowerarm.rod.d_arm, d_rev=lowerarm.rod.d_rev, rho=lowerarm.rod.density, color=lowerarm.rod.color}
      mask prompts: L "Length (m)"; r "Radius (m)"; d_arm "Distance fom center to arm holes (m)"; d_rev "Distance from center to revolute joints (m)"; rho "Density (kg/m^3)"; color "Color [R G B]"
      mask Display: image(fullfile(matlabroot,'toolbox','physmod','sm','smdemos','dump_trailer','images','sm_dump_trailer_rod.png'));
  Center Rod : PMIOPort  Side=Left
  Left Arm Hole : PMIOPort  Port=2  Side=Left
  Left Rod : PMIOPort  Port=3  Side=Left
  Right Arm Hole : PMIOPort  Port=4  Side=Right
  Right Rod : PMIOPort  Port=5  Side=Right
  connections:
  Left Rod/RConn1 -- Rod/LConn2
  Rod/LConn1 -- Left Arm/RConn2
  Left Arm Hole/RConn1 -- Left Arm/RConn1
  Right Arm Hole/RConn1 -- Right Arm/RConn1
  Right Rod/RConn1 -- Rod/RConn2
  Center Rod/RConn1 -- Rod/LConn3
  Rod/RConn1 -- Right Arm/RConn2

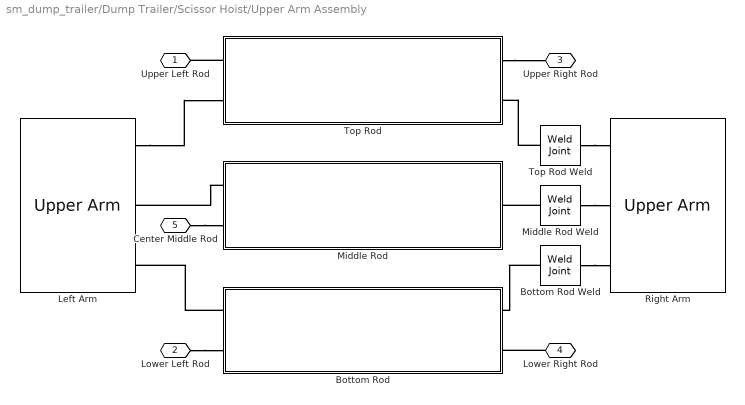
== system sm_dump_trailer/Dump Trailer/Scissor Hoist/Upper Arm Assembly ==
  Bottom Rod : Subsystem  mask{L=upperarm.bottomrod.length, r=upperarm.bottomrod.radius, d_arm=upperarm.bottomrod.d_arm, d_rev=upperarm.bottomrod.d_rev, rho=upperarm.bottomrod.density, color=upperarm.bottomrod.color}
      mask prompts: L "Length (m)"; r "Radius (m)"; d_arm "Distance from center to arm holes (m)"; d_rev "Distance from center to revolute joints (m)"; rho "Density (kg/m^3)"; color "Color [R G B]"
      mask Display: image(fullfile(matlabroot,'toolbox','physmod','sm','smdemos','dump_trailer','images','sm_dump_trailer_rod.png'));
  Bottom Rod Weld : sm_lib/Joints/Weld Joint  JointMode=Normal  SenseConstraintForce=off  SenseConstraintForceX=off  SenseConstraintForceY=off  SenseConstraintForceZ=off  SenseConstraintTorque=off  SenseConstraintTorqueX=off  SenseConstraintTorqueY=off  SenseConstraintTorqueZ=off  SenseTotalForce=off  SenseTotalForceX=off  SenseTotalForceY=off  SenseTotalForceZ=off  SenseTotalTorque=off  SenseTotalTorqueX=off  SenseTotalTorqueY=off  SenseTotalTorqueZ=off  CompositeWrenchDir=FollowerOnBase  CompositeWrenchFrame=BaseFrame
  Left Arm : sm_dump_trailer_lib/Upper Arm  d_top2bot=upperarm.d_bot2top  th_bot2mid=upperarm.th_bot2mid  th_top2mid=upperarm.th_top2mid  T=upperarm.thickness  r_h=upperarm.holeradius  rho=upperarm.density  color=upperarm.color
      settings: SourceProductBaseCode=MS
  Middle Rod : Subsystem  mask{L=upperarm.middlerod.length, r=upperarm.middlerod.radius, d_arm=upperarm.middlerod.d_arm, rho=upperarm.middlerod.density, color=upperarm.middlerod.color}
      mask prompts: L "Length (m)"; r "Radius (m)"; d_arm "Distance from center to arm holes (m)"; rho "Density (kg/m^3)"; color "Color [R G B]"
      mask Display: image(fullfile(matlabroot,'toolbox','physmod','sm','smdemos','dump_trailer','images','sm_dump_trailer_rod.png'));
  Middle Rod Weld : sm_lib/Joints/Weld Joint  JointMode=Normal  SenseConstraintForce=off  SenseConstraintForceX=off  SenseConstraintForceY=off  SenseConstraintForceZ=off  SenseConstraintTorque=off  SenseConstraintTorqueX=off  SenseConstraintTorqueY=off  SenseConstraintTorqueZ=off  SenseTotalForce=off  SenseTotalForceX=off  SenseTotalForceY=off  SenseTotalForceZ=off  SenseTotalTorque=off  SenseTotalTorqueX=off  SenseTotalTorqueY=off  SenseTotalTorqueZ=off  CompositeWrenchDir=FollowerOnBase  CompositeWrenchFrame=BaseFrame
  Right Arm : sm_dump_trailer_lib/Upper Arm  d_top2bot=upperarm.d_bot2top  th_bot2mid=upperarm.th_bot2mid  th_top2mid=upperarm.th_top2mid  T=upperarm.thickness  r_h=upperarm.holeradius  rho=upperarm.density  color=upperarm.color
      settings: SourceProductBaseCode=MS
  Top Rod : Subsystem  mask{L=upperarm.toprod.length, r=upperarm.toprod.radius, d_arm=upperarm.toprod.d_arm, d_rev=upperarm.toprod.d_rev, rho=upperarm.toprod.density, color=upperarm.toprod.color}
      mask prompts: L "Length (m)"; r "Radius (m)"; d_arm "Distance from center to arm holes (m)"; d_rev "Distance from center to revolute joints (m)"; rho "Density (kg/m^3)"; color "Color [R G B]"
      mask Display: image(fullfile(matlabroot,'toolbox','physmod','sm','smdemos','dump_trailer','images','sm_dump_trailer_rod.png'));
  Top Rod Weld : sm_lib/Joints/Weld Joint  JointMode=Normal  SenseConstraintForce=off  SenseConstraintForceX=off  SenseConstraintForceY=off  SenseConstraintForceZ=off  SenseConstraintTorque=off  SenseConstraintTorqueX=off  SenseConstraintTorqueY=off  SenseConstraintTorqueZ=off  SenseTotalForce=off  SenseTotalForceX=off  SenseTotalForceY=off  SenseTotalForceZ=off  SenseTotalTorque=off  SenseTotalTorqueX=off  SenseTotalTorqueY=off  SenseTotalTorqueZ=off  CompositeWrenchDir=FollowerOnBase  CompositeWrenchFrame=BaseFrame
  Upper Left Rod : PMIOPort  Side=Left
  Lower Left Rod : PMIOPort  Port=2  Side=Left
  Upper Right Rod : PMIOPort  Port=3  Side=Right
  Lower Right Rod : PMIOPort  Port=4  Side=Right
  Center Middle Rod : PMIOPort  Port=5  Side=Left
  connections:
  Lower Left Rod/RConn1 -- Bottom Rod/LConn2
  Lower Right Rod/RConn1 -- Bottom Rod/RConn2
  Bottom Rod/LConn1 -- Left Arm/RConn3
  Middle Rod/LConn1 -- Left Arm/RConn2
  Center Middle Rod/RConn1 -- Middle Rod/LConn2
  Left Arm/RConn1 -- Top Rod/LConn2
  Top Rod/LConn1 -- Upper Left Rod/RConn1
  Top Rod/RConn1 -- Upper Right Rod/RConn1
  Middle Rod Weld/LConn1 -- Middle Rod/RConn1
  Middle Rod Weld/RConn1 -- Right Arm/RConn2
  Top Rod Weld/LConn1 -- Top Rod/RConn2
  Top Rod Weld/RConn1 -- Right Arm/RConn1
  Bottom Rod Weld/LConn1 -- Bottom Rod/RConn1
  Bottom Rod Weld/RConn1 -- Right Arm/RConn3

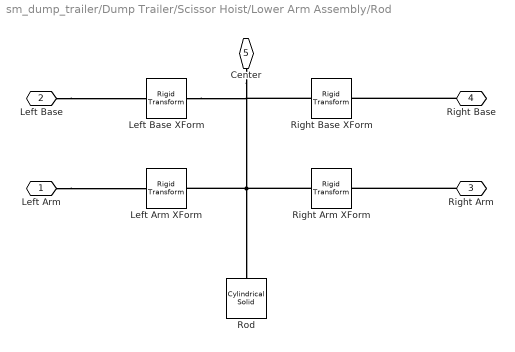
== system sm_dump_trailer/Dump Trailer/Scissor Hoist/Lower Arm Assembly/Rod ==
  Left Arm XForm : sm_lib/Frames and Transforms/Rigid Transform  TranslationMethod=StandardAxis  TranslationStandardOffset=d_arm  TranslationLengthUnit=m  TranslationStandardAxis=-Z  TranslationCartesianOffset=[0 0 0]  TranslationROffset=0  TranslationROffsetUnits=m  TranslationZOffset=0  TranslationZOffsetUnits=m  TranslationThetaOffset=0  TranslationThetaOffsetUnits=deg  RotationMethod=None  RotationAngleUnits=deg  RotationStandardAxis=+Z  RotationAngle=0.0  RotationArbitraryAxis=[0 0 1]  FollAlignAxisA=+X  BaseAlignAxisA=+Y  FollAlignAxisB=+Y  BaseAlignAxisB=+Z  RotationSequenceAxes=FollowerAxes  RotationSequence=XYX  RotationSequenceAngles=[0 0 0]  RotationSequenceAnglesUnits=deg  RotationMatrix=[1 0 0; 0 1 0; 0 0 1]
  Left Base XForm : sm_lib/Frames and Transforms/Rigid Transform  TranslationMethod=StandardAxis  TranslationStandardOffset=d_rev  TranslationLengthUnit=m  TranslationStandardAxis=-Z  TranslationCartesianOffset=[0 0 0]  TranslationROffset=0  TranslationROffsetUnits=m  TranslationZOffset=0  TranslationZOffsetUnits=m  TranslationThetaOffset=0  TranslationThetaOffsetUnits=deg  RotationMethod=None  RotationAngleUnits=deg  RotationStandardAxis=+Z  RotationAngle=0.0  RotationArbitraryAxis=[0 0 1]  FollAlignAxisA=+X  BaseAlignAxisA=+Y  FollAlignAxisB=+Y  BaseAlignAxisB=+Z  RotationSequenceAxes=FollowerAxes  RotationSequence=XYX  RotationSequenceAngles=[0 0 0]  RotationSequenceAnglesUnits=deg  RotationMatrix=[1 0 0; 0 1 0; 0 0 1]
  Right Arm XForm : sm_lib/Frames and Transforms/Rigid Transform  TranslationMethod=StandardAxis  TranslationStandardOffset=d_arm  TranslationLengthUnit=m  TranslationStandardAxis=+Z  TranslationCartesianOffset=[0 0 0]  TranslationROffset=0  TranslationROffsetUnits=m  TranslationZOffset=0  TranslationZOffsetUnits=m  TranslationThetaOffset=0  TranslationThetaOffsetUnits=deg  RotationMethod=None  RotationAngleUnits=deg  RotationStandardAxis=+Z  RotationAngle=0.0  RotationArbitraryAxis=[0 0 1]  FollAlignAxisA=+X  BaseAlignAxisA=+Y  FollAlignAxisB=+Y  BaseAlignAxisB=+Z  RotationSequenceAxes=FollowerAxes  RotationSequence=XYX  RotationSequenceAngles=[0 0 0]  RotationSequenceAnglesUnits=deg  RotationMatrix=[1 0 0; 0 1 0; 0 0 1]
  Right Base XForm : sm_lib/Frames and Transforms/Rigid Transform  TranslationMethod=StandardAxis  TranslationStandardOffset=d_rev  TranslationLengthUnit=m  TranslationStandardAxis=+Z  TranslationCartesianOffset=[0 0 0]  TranslationROffset=0  TranslationROffsetUnits=m  TranslationZOffset=0  TranslationZOffsetUnits=m  TranslationThetaOffset=0  TranslationThetaOffsetUnits=deg  RotationMethod=None  RotationAngleUnits=deg  RotationStandardAxis=+Z  RotationAngle=0.0  RotationArbitraryAxis=[0 0 1]  FollAlignAxisA=+X  BaseAlignAxisA=+Y  FollAlignAxisB=+Y  BaseAlignAxisB=+Z  RotationSequenceAxes=FollowerAxes  RotationSequence=XYX  RotationSequenceAngles=[0 0 0]  RotationSequenceAnglesUnits=deg  RotationMatrix=[1 0 0; 0 1 0; 0 0 1]
  Rod : sm_lib/Body Elements/Cylindrical Solid  GraphicAmbientColor=[0.15 0.15 0.15 1.0]  BasedOnType=Density  CenterOfMass=[0 0 0]  CenterOfMassUnits=m  GraphicDiffuseColor=color  CylinderLength=L  CylinderLengthUnits=m  CylinderRadius=r  CylinderRadiusUnits=m  Density=rho  DensityUnits=kg/m^3  DoExposeReferenceFrame=on  GraphicEmissiveColor=[0.0 0.0 0.0 1.0]  ExportEntireGeometry=off  SerializedFrames=<Frames/>  MarkerShape=Sphere  MarkerSize=10  GraphicType=FromGeometry  InertiaType=CalculateFromGeometry  Mass=1  MassUnits=kg  MomentsOfInertia=[1 1 1]  MomentsOfInertiaUnits=kg*m^2  GraphicOpacity=1.0  ProductsOfInertia=[1 1 1]  ProductsOfInertiaUnits=kg*m^2  GraphicShininess=75  GraphicSpecularColor=[0.5 0.5 0.5 1.0]  GraphicVisPropType=SimpleVisualProperties
  Left Arm : PMIOPort  Side=Left
  Left Base : PMIOPort  Port=2  Side=Left
  Right Arm : PMIOPort  Port=3  Side=Right
  Right Base : PMIOPort  Port=4  Side=Right
  Center : PMIOPort  Port=5  Side=Left
  connections:
  Right Arm XForm/LConn1 -- Center/RConn1 -- Right Base XForm/LConn1 -- Left Base XForm/LConn1 -- Left Arm XForm/LConn1 -- Rod/RConn1
  Left Base/RConn1 -- Left Base XForm/RConn1
  Left Arm/RConn1 -- Left Arm XForm/RConn1
  Right Base/RConn1 -- Right Base XForm/RConn1
  Right Arm/RConn1 -- Right Arm XForm/RConn1

== system sm_dump_trailer/Dump Trailer/Scissor Hoist/Upper Arm Assembly/Bottom Rod ==
  Left Arm XForm : sm_lib/Frames and Transforms/Rigid Transform  TranslationMethod=StandardAxis  TranslationStandardOffset=d_arm  TranslationLengthUnit=m  TranslationStandardAxis=-Z  TranslationCartesianOffset=[0 0 0]  TranslationROffset=0  TranslationROffsetUnits=m  TranslationZOffset=0  TranslationZOffsetUnits=m  TranslationThetaOffset=0  TranslationThetaOffsetUnits=deg  RotationMethod=None  RotationAngleUnits=deg  RotationStandardAxis=+Z  RotationAngle=0.0  RotationArbitraryAxis=[0 0 1]  FollAlignAxisA=+X  BaseAlignAxisA=+Y  FollAlignAxisB=+Y  BaseAlignAxisB=+Z  RotationSequenceAxes=FollowerAxes  RotationSequence=XYX  RotationSequenceAngles=[0 0 0]  RotationSequenceAnglesUnits=deg  RotationMatrix=[1 0 0; 0 1 0; 0 0 1]
  Left Revolute XForm : sm_lib/Frames and Transforms/Rigid Transform  TranslationMethod=StandardAxis  TranslationStandardOffset=d_rev  TranslationLengthUnit=m  TranslationStandardAxis=-Z  TranslationCartesianOffset=[0 0 0]  TranslationROffset=0  TranslationROffsetUnits=m  TranslationZOffset=0  TranslationZOffsetUnits=m  TranslationThetaOffset=0  TranslationThetaOffsetUnits=deg  RotationMethod=None  RotationAngleUnits=deg  RotationStandardAxis=+Z  RotationAngle=0.0  RotationArbitraryAxis=[0 0 1]  FollAlignAxisA=+Z  BaseAlignAxisA=-Z  FollAlignAxisB=+Y  BaseAlignAxisB=+Y  RotationSequenceAxes=FollowerAxes  RotationSequence=XYX  RotationSequenceAngles=[0 0 0]  RotationSequenceAnglesUnits=deg  RotationMatrix=[1 0 0; 0 1 0; 0 0 1]
  Right Arm XForm : sm_lib/Frames and Transforms/Rigid Transform  TranslationMethod=StandardAxis  TranslationStandardOffset=d_arm  TranslationLengthUnit=m  TranslationStandardAxis=+Z  TranslationCartesianOffset=[0 0 0]  TranslationROffset=0  TranslationROffsetUnits=m  TranslationZOffset=0  TranslationZOffsetUnits=m  TranslationThetaOffset=0  TranslationThetaOffsetUnits=deg  RotationMethod=None  RotationAngleUnits=deg  RotationStandardAxis=+Z  RotationAngle=0.0  RotationArbitraryAxis=[0 0 1]  FollAlignAxisA=+X  BaseAlignAxisA=+Y  FollAlignAxisB=+Y  BaseAlignAxisB=+Z  RotationSequenceAxes=FollowerAxes  RotationSequence=XYX  RotationSequenceAngles=[0 0 0]  RotationSequenceAnglesUnits=deg  RotationMatrix=[1 0 0; 0 1 0; 0 0 1]
  Right Revolute XForm : sm_lib/Frames and Transforms/Rigid Transform  TranslationMethod=StandardAxis  TranslationStandardOffset=d_rev  TranslationLengthUnit=m  TranslationStandardAxis=+Z  TranslationCartesianOffset=[0 0 0]  TranslationROffset=0  TranslationROffsetUnits=m  TranslationZOffset=0  TranslationZOffsetUnits=m  TranslationThetaOffset=0  TranslationThetaOffsetUnits=deg  RotationMethod=None  RotationAngleUnits=deg  RotationStandardAxis=+Z  RotationAngle=0.0  RotationArbitraryAxis=[0 0 1]  FollAlignAxisA=+Z  BaseAlignAxisA=-Z  FollAlignAxisB=+Y  BaseAlignAxisB=+Y  RotationSequenceAxes=FollowerAxes  RotationSequence=XYX  RotationSequenceAngles=[0 0 0]  RotationSequenceAnglesUnits=deg  RotationMatrix=[1 0 0; 0 1 0; 0 0 1]
  Rod : sm_lib/Body Elements/Cylindrical Solid  GraphicAmbientColor=[0.15 0.15 0.15 1.0]  BasedOnType=Density  CenterOfMass=[0 0 0]  CenterOfMassUnits=m  GraphicDiffuseColor=color  CylinderLength=L  CylinderLengthUnits=m  CylinderRadius=r  CylinderRadiusUnits=m  Density=rho  DensityUnits=kg/m^3  DoExposeReferenceFrame=on  GraphicEmissiveColor=[0.0 0.0 0.0 1.0]  ExportEntireGeometry=off  SerializedFrames=<Frames/>  MarkerShape=Sphere  MarkerSize=10  GraphicType=FromGeometry  InertiaType=CalculateFromGeometry  Mass=1  MassUnits=kg  MomentsOfInertia=[1 1 1]  MomentsOfInertiaUnits=kg*m^2  GraphicOpacity=1.0  ProductsOfInertia=[1 1 1]  ProductsOfInertiaUnits=kg*m^2  GraphicShininess=75  GraphicSpecularColor=[0.5 0.5 0.5 1.0]  GraphicVisPropType=SimpleVisualProperties
  Left Arm : PMIOPort  Side=Left
  Left Revolute : PMIOPort  Port=2  Side=Left
  Right Arm : PMIOPort  Port=3  Side=Right
  Right Revolute : PMIOPort  Port=4  Side=Right
  connections:
  Right Revolute XForm/LConn1 -- Left Arm XForm/LConn1 -- Rod/RConn1 -- Right Arm XForm/LConn1 -- Left Revolute XForm/LConn1
  Left Revolute/RConn1 -- Left Revolute XForm/RConn1
  Left Arm/RConn1 -- Left Arm XForm/RConn1
  Right Revolute/RConn1 -- Right Revolute XForm/RConn1
  Right Arm/RConn1 -- Right Arm XForm/RConn1
